simulink subsystem "TwoPhaseModification"  (R2021b)
settings: Solver=VariableStepAuto  StartTime=0.0  StopTime=10.0  RelTol=1e-3
libraries: fl_lib x6, nesl_utility x1
settings Model: Creator=silen  LastModifiedBy=Jiaqi

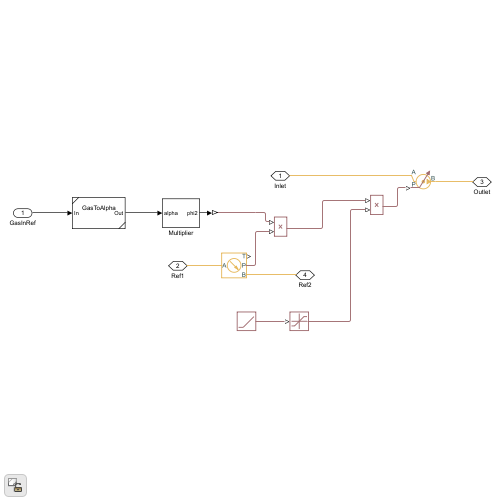
[thumbnail: Simulink's stored preview of the top-level diagram]
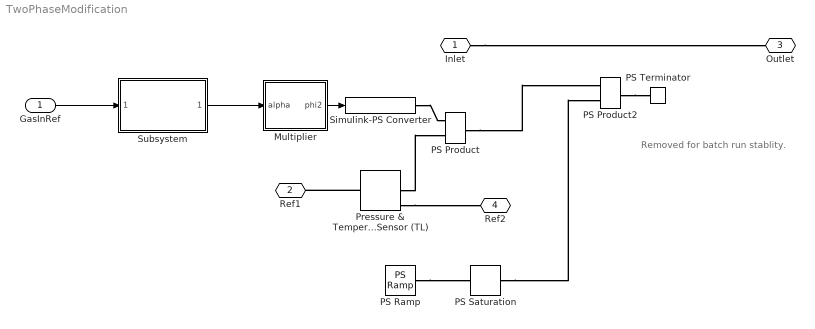
== system TwoPhaseModification ==
  note: Removed for batch run stablity.
  GasInRef : Inport
  Multiplier : Subsystem
  PS Product : fl_lib/Physical Signals/Functions/PS Product
  PS Product2 : fl_lib/Physical Signals/Functions/PS Product
  PS Ramp : fl_lib/Physical Signals/Sources/PS Ramp  slope=0.1 1/s  start_time=30 s  initial_output=0
      settings: SourceProductBaseCode=SS
  PS Saturation : fl_lib/Physical Signals/Nonlinear Operators/PS Saturation  upper_limit=1  lower_limit=0
      settings: SourceProductBaseCode=SS
  PS Terminator : fl_lib/Physical Signals/Sinks/PS Terminator
  Pressure & Temperature Sensor (TL) : fl_lib/Thermal Liquid/Sensors/Pressure & Temperature Sensor (TL)
      settings: SourceProductBaseCode=SS  InternalSimscapePortConfiguration="{\"Bottom\":[],\"Left\":[{\"id\":\"A\",\"label\":\"A\",\"type\":\"foundation.thermal_liquid.thermal_liquid\"}],\"Right\":[{\"id\":\"B\",\"label\":\"B\",\"type\":\"foundation.thermal_liquid.thermal_liquid\"},{\"id\":\"P\",\"label\":\"P\",\"type\":\"output\"},{\"id\":\"T\",\"label\":\"T\",\"type\":\"output\"}],\"Top\":[]}"
  Simulink-PS Converter : nesl_utility/Simulink-PS Converter  PhysicalDomain=network_engine_domain  SubClassName=ps_input  LeftPortType=input  RightPortType=output  PseudoPeriodic=off  Frequencies=[]  NoiseDistribution=none  NoiseParameters=[]  Unit=1  AffineConversion=off  FilteringAndDerivatives=provide  SimscapeFilterOrder=1  InputFilterTimeConstant=0.001  UdotUserProvided=0
      settings: SourceProductBaseCode=PW,SS
  Subsystem : Subsystem  ReferencedSubsystem=GasToAlpha
  Inlet : PMIOPort  Side=Left
  Ref1 : PMIOPort  Port=2  Side=Left
  Outlet : PMIOPort  Port=3  Side=Right
  Ref2 : PMIOPort  Port=4  Side=Right
  wires:
  GasInRef/1 -> Subsystem/1
  Multiplier/1(phi2) -> Simulink-PS Converter/1
  Subsystem/1 -> Multiplier/1(alpha)
  connections:
  Pressure & Temperature Sensor (TL)/RConn1 -- Ref2/RConn1
  Inlet/RConn1 -- Outlet/RConn1
  Pressure & Temperature Sensor (TL)/LConn1 -- Ref1/RConn1
  Simulink-PS Converter/RConn1 -- PS Product/LConn1
  Pressure & Temperature Sensor (TL)/RConn2 -- PS Product/LConn2
  PS Product/RConn1 -- PS Product2/LConn1
  PS Saturation/RConn1 -- PS Product2/LConn2
  PS Ramp/RConn1 -- PS Saturation/LConn1
  PS Product2/RConn1 -- PS Terminator/LConn1

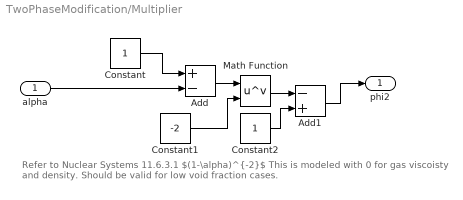
== system TwoPhaseModification/Multiplier ==
  note: Refer to Nuclear Systems 11.6.3.1
      | $(1-\alpha)^{-2}$
      | This is modeled with 0 for gas viscoisty and density. Should be valid for low void fraction cases.
  alpha : Inport
  Add : Sum  Inputs=+-
  Add1 : Sum  Inputs=-+
  Constant : Constant
  Constant1 : Constant  Value=-2
  Constant2 : Constant
  Math Function : Math  Operator=pow  SaturateOnIntegerOverflow=on
  phi2 : Outport
  wires:
  Add1/1 -> phi2/1
  Constant/1 -> Add/1
  alpha/1 -> Add/2
  Add/1 -> Math Function/1
  Constant2/1 -> Add1/2
  Constant1/1 -> Math Function/2
  Math Function/1 -> Add1/1
